simulink model "control_inverted_pendulum"  (R2025a)
settings: Solver=FixedStepAuto  StartTime=0.0  StopTime=5  FixedStep=1.0e-5  RelTol=1e-3
undefined symbols (not defined in the file): p_btheta, p_bx, p_Dz, p_G, p_g, p_Iw, p_Jp, p_Ke, p_Kt, p_l, p_La, p_M, p_m, p_r, p_Ra
libraries: mpclib x1
settings Model: Creator=nopla  LastModifiedBy=nop
settings OptimizationCC: UseDivisionForNetSlopeComputation=on

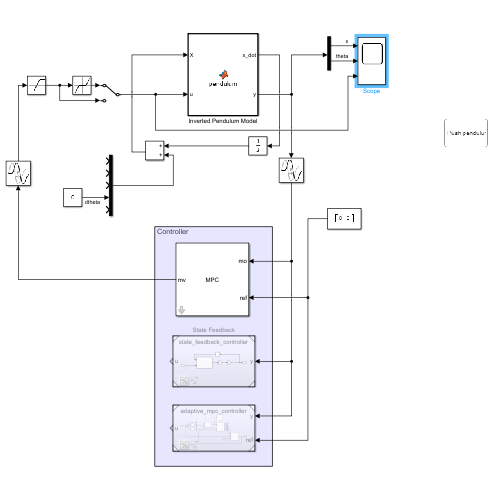
[thumbnail: Simulink's stored preview of the top-level diagram]
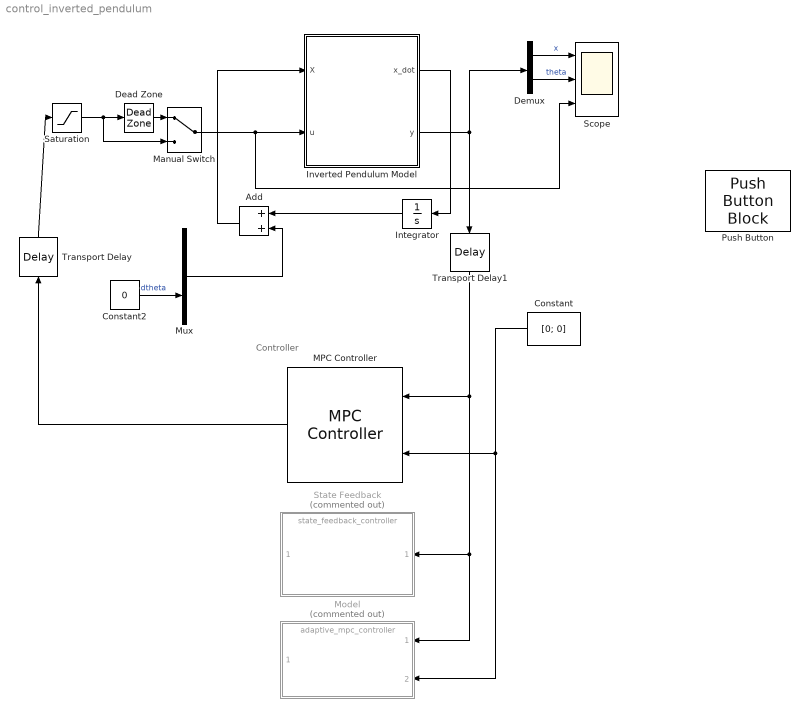
== system control_inverted_pendulum ==
  note: Controller
  Add : Sum
  Constant : Constant  Value=[0; 0]
  Constant2 : Constant  Value=0
  Dead Zone : DeadZone  LowerValue=-p_Dz  UpperValue=p_Dz
  Demux : Demux  Outputs=2
  Integrator : Integrator  InitialCondition=[0; 0; 0.01; 0; 0]
  Inverted Pendulum Model : MATLAB Function  TreatAsAtomicUnit=on
  MPC Controller : mpclib/MPC Controller  SCDEnableBlockLinearizationSpecification=on  mpcobj=mpcobj  is_multiple=0  enable_value=0  return_u0=off  updateMPCinCallerWorkspace=on  md_inport=off  mv_inport=off  uref_inport=off  return_cost=off  return_mvseq=off  return_qpstatus=off  return_xseq=off  return_state=off  return_ovseq=off  state_inport=off  umin_inport=off  umax_inport=off  ymin_inport=off  ymax_inport=off  cc_inport=off  ywt_inport=off  uwt_inport=off  duwt_inport=off  rhoeps_inport=off  pm_inport=off  MaximumP=10  HorizonChoice=FixedHorizon  n_ts=0.01  n_p=100  n_mv=1  n_md=0  n_ud=0  n_mo=2  n_uo=0  BlockDataType=double  SampleTimeInherited=off  switch_inport=off
  Manual Switch : ManualSwitch
  Model : ModelReference  Commented=on  ModelNameDialog=adaptive_mpc_controller.slx  SimulationMode=Normal  ModelReferenceVersion=1.25
  Mux : Mux  Inputs=5
  Push Button : PushButtonBlock  ButtonText=Push pendulum  OnValue=0.1  IconOnColor=[0.0, 0.39215686274509803, 0.0]  IconOffColor=[0.0, 1.0, 0.0]  OffValue=0.000000
  Saturation : Saturate  UpperLimit=7.2  LowerLimit=-7.2
  Scope : Scope  NumInputPorts=3
      settings: ActiveDisplayYMinimum=-5.8937131998808878  ActiveDisplayYMaximum=5.0579911970660145  DataLoggingVariableName=ScopeData2  DataLoggingSaveFormat=Array
  State Feedback : ModelReference  Commented=on  ModelNameDialog=state_feedback_controller.slx  SimulationMode=Normal  ModelReferenceVersion=1.193
  Transport Delay : TransportDelay  DelayTime=0.001
  Transport Delay1 : TransportDelay  DelayTime=0
  wires:
  Inverted Pendulum Model/1(x_dot) -> Integrator/1
  Integrator/1 -> Add/1
  Demux/1 -> Scope/1  "x"
  Demux/2 -> Scope/2  "theta"
  Inverted Pendulum Model/2(y) -> Demux/1, Transport Delay1/1
  Constant/1 -> MPC Controller/2, Model/2
  Transport Delay1/1 -> MPC Controller/1, State Feedback/1, Model/1
  Transport Delay/1 -> Saturation/1
  Add/1 -> Inverted Pendulum Model/1(X)
  Mux/1 -> Add/2
  Constant2/1 -> Mux/4  "dtheta"
  Saturation/1 -> Manual Switch/2, Dead Zone/1
  Manual Switch/1 -> Inverted Pendulum Model/2(u), Scope/3
  Dead Zone/1 -> Manual Switch/1
  MPC Controller/1 -> Transport Delay/1

== matlab function control_inverted_pendulum/Inverted Pendulum Model ==
  data: x_dot output size=[5 1]; y output; X input size=[5 1]; u input; p_M parameter; p_m parameter; p_g parameter; p_l parameter; p_r parameter; p_Iw parameter; p_G parameter; p_Jp parameter; p_bx parameter; p_btheta parameter; p_Kt parameter; p_Ke parameter; p_Ra parameter; p_La parameter
function [x_dot, y] = pendulum(X, u, p_M, p_m, p_g, p_l, p_r, p_Iw, p_G, p_Jp, p_bx, p_btheta, p_Kt, p_Ke, p_Ra, p_La)
% 台車型倒立振子の状態空間動力学
% 
% 入力:
%   X: 状態ベクトル [x; x_dot; theta; theta_dot; i] (5x1)
%   u: 入力電圧 V (スカラー)
%   params: パラメータ構造体

params = [p_M; p_m; p_g; p_l; p_r; p_Iw; p_G; p_Jp; p_bx; p_btheta; p_Kt; p_Ke; p_Ra; p_La];

x_dot = nonlinear_dynamics(X, u, params);

y = [X(1); X(3)];

end
